simulink model "Consensus_Demo_01_configuration"  (R2021b)
settings: Solver=VariableStepAuto  StartTime=0.0  StopTime=10.0  RelTol=1e-3
model workspace (MAT data in the model file):
  x1 = 1
libraries: simulink x1
settings Model: Creator=vijay  LastModifiedBy=vijay

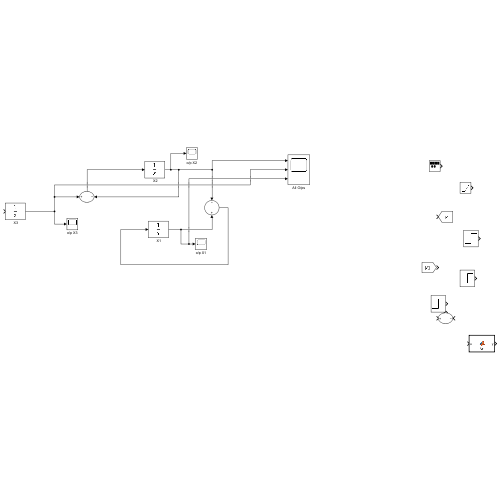
[thumbnail: Simulink's stored preview of the top-level diagram]
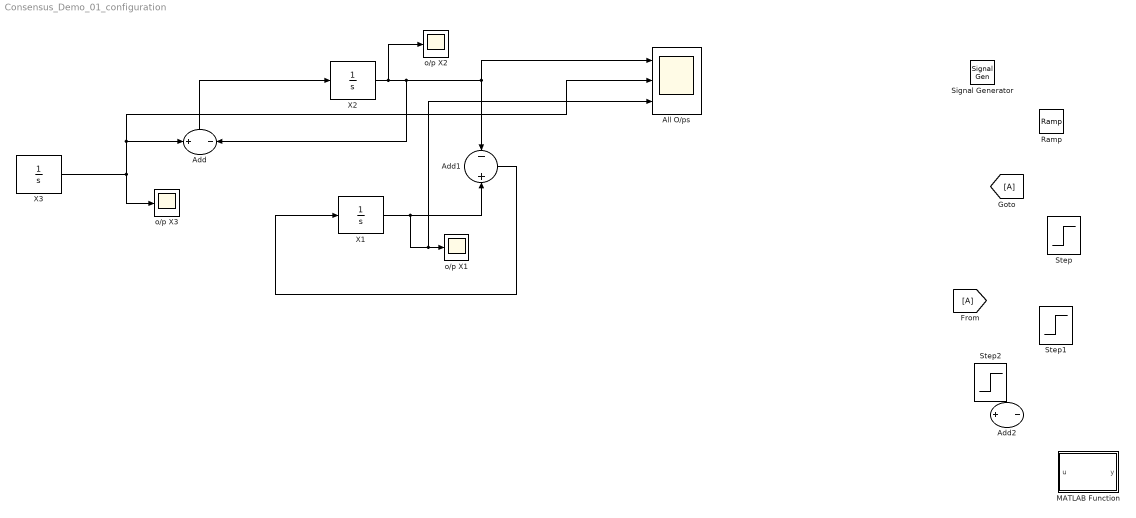
== system Consensus_Demo_01_configuration ==
  " X1" : Integrator  InitialCondition=0.2
  " X2" : Integrator  InitialCondition=0.4
  " X3" : Integrator  InitialCondition=0.6
  Add : Sum  Inputs=+-
  Add1 : Sum  Inputs=-+
  Add2 : Sum  Inputs=+-
  All O/ps : Scope  NumInputPorts=3
  MATLAB Function : MATLAB Function  TreatAsAtomicUnit=on
  Ramp : simulink/Sources/Ramp  slope=1  start=0  InitialOutput=0
  Signal Generator : SignalGenerator  WaveForm=random  Units=rad/sec
  Step : Step  SampleTime=0
  Step1 : Step  SampleTime=0
  Step2 : Step  SampleTime=0
  o/p X1 : Scope
  o/p X2 : Scope
  o/p X3 : Scope
  wires:
  Add/1 -> " X2"/1
  " X2"/1 -> o/p X2/1, Add/2, Add1/1, All O/ps/1
  " X1"/1 -> All O/ps/3, o/p X1/1, Add1/2
  Add1/1 -> " X1"/1
  " X3"/1 -> All O/ps/2, Add/1, o/p X3/1

== matlab function Consensus_Demo_01_configuration/MATLAB Function ==
  data: u input; y output
function y = fcn(u)

y = u;
